simulink model "modeltest_model"  (Simulink 8.5)
settings: Solver=ode1  StartTime=0.0  StopTime=5  FixedStep=0.01  RelTol=1e-3
undefined symbols (not defined in the file or in its folder): a, pmax
settings Model: Creator=nogueira_raf  LastModifiedBy=nogueira_raf
settings DataIOCC: InitialState=2000  SignalLoggingSaveFormat=Dataset  SaveOutput=off  SaveTime=off
settings OptimizationCC: BooleanDataType=off  ExpressionDepthLimit=128
settings DebuggingCC: UnderspecifiedInitializationDetection=Simplified  MergeDetectMultiDrivingBlocksExec=error  FcnCallInpInsideContextMsg=EnableAllAsError  StateNameClashWarn=none
settings GRTTargetCC: CombineOutputUpdateFcns=on  GRTInterface=off

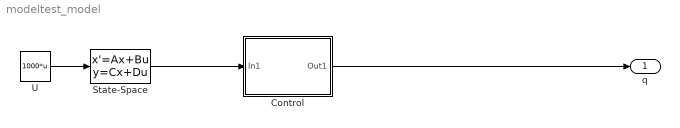
== system modeltest_model ==
  Control : Subsystem
  State-Space : StateSpace  A=-1/a  B=1/a  D=0  X0=20000
  U : Constant  Value=1000*u
  q : Outport
  wires:
  U/1 -> State-Space/1
  State-Space/1 -> Control/1(In1)
  Control/1(Out1) -> q/1

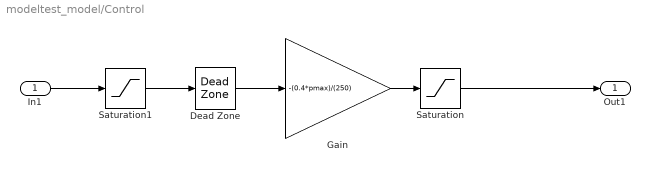
== system modeltest_model/Control ==
  In1 : Inport
  Dead Zone : DeadZone  LowerValue=19250  UpperValue=20750  SaturateOnIntegerOverflow=on
  Gain : Gain  Gain=-(0.4*pmax)/(250)
  Saturation : Saturate  UpperLimit=0.4*pmax  LowerLimit=-0.4*pmax
  Saturation1 : Saturate  UpperLimit=21000  LowerLimit=18000
  Out1 : Outport
  wires:
  Gain/1 -> Saturation/1
  In1/1 -> Saturation1/1
  Dead Zone/1 -> Gain/1
  Saturation1/1 -> Dead Zone/1
  Saturation/1 -> Out1/1
